simulink model "stepRecovery_compatibility"  (Simulink 8.3)
settings: Solver=ode3  SolverMode=SingleTasking  StartTime=0.0  StopTime="CONFIG.SIMULATION_TIME "  FixedStep=CONFIG.Ts  RelTol=1e-3
InitFcn:
  | cd(fileparts(which(bdroot)));
  | initStepRecovery;
values from neighbouring files (symbols this model uses):
  baseToWorldRotationPort = '/matlabTorqueBalancing/floatingBaseRotationMatrix:i'    [esperimento_fake2.mat]    (also in initStepRecovery.m = ['/' WBT_modelName '/floatingBaseRotationMatrix:i']; initTorqueBalancing.m = ['/' WBT_modelName '/floatingBaseRotationMatrix:i']; secondo_risultato.mat)
  bVectorConstraints = [0 0 0 0 0 0 0 0 0 0 0 0 ... (19 elements, 19x1)]    [esperimento_fake2.mat]    (also in secondo_risultato.mat)
  CONFIG =     [esperimento_fake2.mat]    (also in secondo_risultato.mat)
  ConstraintsMatrix = [3.73205080757 1 0.267949192431 -0.267949192431 -1 -3.73205080757 -3.73205080757 -1 -0.267949192431 0.267949192431 1 3.73205080757 ... (114 elements, 19x6)]    [esperimento_fake2.mat]    (also in secondo_risultato.mat)
  gain =     [esperimento_fake2.mat]    (also in secondo_risultato.mat)
  references =     [esperimento_fake2.mat]    (also in secondo_risultato.mat)
  reg =     [esperimento_fake2.mat]    (also in secondo_risultato.mat)
  ROBOT_DOF = 23    [esperimento_fake2.mat]    (also in secondo_risultato.mat)
  ROBOT_DOF_FOR_SIMULINK = [1 0 0 0 0 0 0 0 0 0 0 0 ... (529 elements, 23x23)]    [esperimento_fake2.mat]    (also in secondo_risultato.mat)
  sat =     [esperimento_fake2.mat]    (also in secondo_risultato.mat)
  SM =     [esperimento_fake2.mat]    (also in secondo_risultato.mat)
  sm =     [esperimento_fake2.mat]    (also in secondo_risultato.mat)
  WBT_modelName = 'matlabTorqueBalancing'    [esperimento_fake2.mat]    (also in initStepRecovery.m; initTorqueBalancing.m; secondo_risultato.mat)
  WBT_robotName = ''    [esperimento_fake2.mat]    (also in secondo_risultato.mat)
undefined symbols (not defined in the file or in its folder): bVectorConstraintsMPC, ConstraintsMatrixMPC, DiscIntNeverNeededParam, mpc_init
libraries: WBToolboxLibrary x191, simulink x22, simulink_extras x4
(part 4 of 6)

== system stepRecovery_compatibility/DesValues/State Machine/visualise inertial/w_H_root_link4 ==
  qj : Inport
  inertial : Inport  Port=2
  "CoM6D ->  CoMXYZ1" : Selector  NumberOfDimensions=2  InputPortWidth=7  IndexOptions=Index vector (dialog),Index vector (dialog)  Indices=[1 2 3],[1 2 3]  OutputSizes=1,1
  Constant : Constant  Value=zeros(3,1)
  Constant2 : Constant  Value=eye(4)
  Constant5 : Constant  Value=eye(4)
  Constant6 : Constant  Value=eye(4)
  Gain : Gain  Gain=pi/180
  Head state : WBToolboxLibrary/Utilities/Yarp Read  portName=[WBT_robotName, '/head/state:o']  signalSize=6  blocking=off  timestamp=off  autoconnect=on  errorOnConnection=off
  Inv\* : Product  Inputs=/*  Multiplication=Matrix(*)
  Inv\*1 : Product  Inputs=/*  Multiplication=Matrix(*)
  Inv\*2 : Product  Inputs=/  Multiplication=Matrix(*)
  Product : Product  Multiplication=Matrix(*)
  Selector : Selector  InputPortWidth=12  IndexOptions=Index vector (dialog)  Indices=[4 5 6 ]  OutputSizes=1
  Selector1 : Selector  InputPortWidth=6  IndexOptions=Index vector (dialog)  Indices=[1:3]  OutputSizes=1
  Switch : Switch  Criteria=u2 > Threshold
  Switch6 : Switch  Criteria=u2 > Threshold
  USE_IMU4EST_BASE : Constant  Value=CONFIG.USE_IMU4EST_BASE
  USE_IMU4EST_BASE1 : Constant  Value=CONFIG.CORRECT_NECK_IMU
  fromImuToHomogeousTransformFCN : MATLAB Function  TreatAsAtomicUnit=on
      settings: PermitHierarchicalResolution=ParametersOnly
  holder 1 : WBToolboxLibrary/Utilities/holder 
  holder 2 : WBToolboxLibrary/Utilities/holder 
  imu : WBToolboxLibrary/wholeBodyModel/Kinematics/Forward Kinematics  frameName='imu_frame'  robotName=WBT_robotName  localName=WBT_modelName  wbiFile=WBT_wbiFilename  wbiList=WBT_wbiList
  l_sole_acc : Scope
      settings: TimeRange=60  ShowLegends=on  MaxDataPoints=5000  SaveToWorkspace=off  YMin=-4.47309  YMax=14.2668  SampleTime=-1
  link : WBToolboxLibrary/wholeBodyModel/Kinematics/Forward Kinematics  frameName=link_name  robotName=WBT_robotName  localName=WBT_modelName  wbiFile=WBT_wbiFilename  wbiList=WBT_wbiList
  root_link : WBToolboxLibrary/wholeBodyModel/Kinematics/Forward Kinematics  frameName='root_link'  robotName=WBT_robotName  localName=WBT_modelName  wbiFile=WBT_wbiFilename  wbiList=WBT_wbiList
  w_H_root : Outport
  wires:
  Constant5/1 -> imu/1
  Inv\*/1 -> Inv\*2/1, holder 1/1, fromImuToHomogeousTransformFCN/1(imu_H_link)  "imu_H_link"
  imu/1 -> Inv\*/1
  Constant6/1 -> link/1
  Inv\*1/1 -> Switch6/3, fromImuToHomogeousTransformFCN/3(link_H_root)  "link_H_root"
  link/1 -> Inv\*/2, Inv\*1/1
  inertial/1 -> Selector/1, holder 2/1, fromImuToHomogeousTransformFCN/5(inertial)
  Switch6/1 -> w_H_root/1
  USE_IMU4EST_BASE/1 -> Switch6/2
  fromImuToHomogeousTransformFCN/1(w_H_root) -> Switch6/1
  Constant2/1 -> root_link/1
  qj/1 -> root_link/2, link/2, imu/2
  root_link/1 -> Inv\*1/2
  holder 1/1 -> fromImuToHomogeousTransformFCN/2(imu_H_link_0)
  holder 2/1 -> fromImuToHomogeousTransformFCN/4(inertial_0)
  Inv\*2/1 -> "CoM6D ->  CoMXYZ1"/1
  "CoM6D ->  CoMXYZ1"/1 -> Product/1  "l_sole_R_imu"
  Selector/1 -> Product/2  "imu_acce"
  Product/1 -> l_sole_acc/1
  Head state/1 -> Gain/1
  Selector1/1 -> Switch/1  "neck"
  USE_IMU4EST_BASE1/1 -> Switch/2
  Switch/1 -> fromImuToHomogeousTransformFCN/6(neck)
  Gain/1 -> Selector1/1
  Constant/1 -> Switch/3

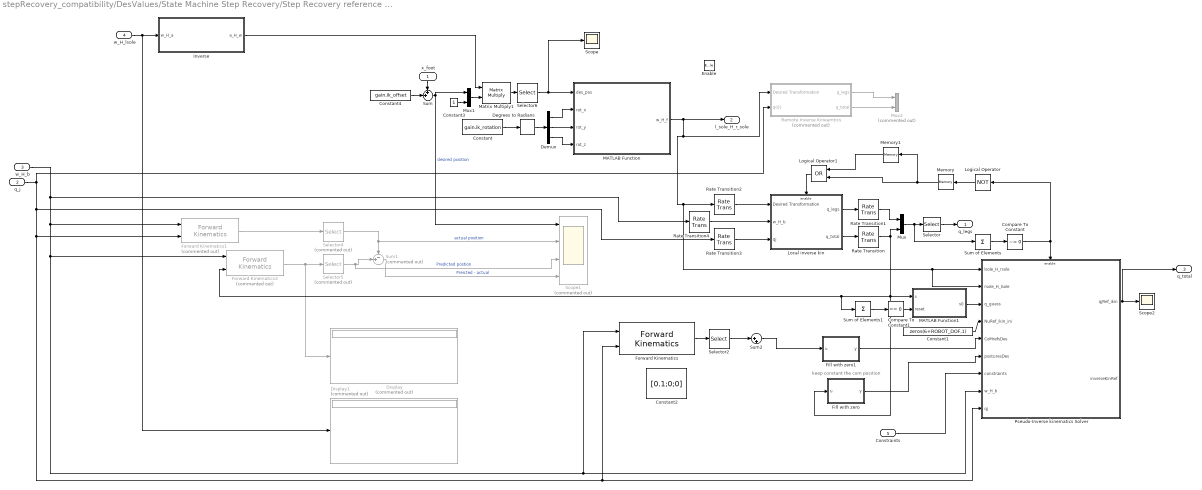
== system stepRecovery_compatibility/DesValues/State Machine Step Recovery/Step Recovery reference generator/Inverse Kinematics ==
  note: keep constant the com position
  x_foot : Inport
  q_j : Inport  Port=2
  w_H_b : Inport  Port=3
  w_H_lsole : Inport  Port=4
  Constraints : Inport  Port=5
  Enable : EnablePort
  Compare To Constant : simulink/Logic and Bit Operations/Compare To Constant  relop=~=  const=0  OutDataTypeStr=boolean
  Compare To Constant1 : simulink/Logic and Bit Operations/Compare To Constant  relop===  const=0  OutDataTypeStr=boolean
  Constant : Constant  Value=gain.ik_rotation
  Constant1 : Constant  Value=zeros(6+ROBOT_DOF,1)
  Constant2 : Constant  Value=[0.1;0;0]
  Constant3 : Constant
  Constant4 : Constant  Value=gain.ik_offset
  Degrees to Radians : simulink_extras/Transformations/Degrees to Radians
  Demux : Demux  Outputs=3
  Display : Display  Commented=on
  Display1 : Display  Commented=on
  Fill with zero : MATLAB Function  TreatAsAtomicUnit=on
      settings: PermitHierarchicalResolution=ParametersOnly
  Fill with zero1 : MATLAB Function  TreatAsAtomicUnit=on
      settings: PermitHierarchicalResolution=ParametersOnly
  Forward Kinematics : WBToolboxLibrary/wholeBodyModel/Kinematics/Forward Kinematics  frameName='com'  robotName=WBT_robotName  localName=WBT_modelName  wbiFile=WBT_wbiFilename  wbiList=WBT_wbiList
  Forward Kinematics1 : WBToolboxLibrary/wholeBodyModel/Kinematics/Forward Kinematics  Commented=on  frameName='r_sole'  robotName=WBT_robotName  localName=WBT_modelName  wbiFile=WBT_wbiFilename  wbiList=WBT_wbiList
  Forward Kinematics3 : WBToolboxLibrary/wholeBodyModel/Kinematics/Forward Kinematics  Commented=on  frameName='r_sole'  robotName=WBT_robotName  localName=WBT_modelName  wbiFile=WBT_wbiFilename  wbiList=WBT_wbiList
  Inverse : MATLAB Function  TreatAsAtomicUnit=on
      settings: PermitHierarchicalResolution=ParametersOnly
  Local inverse kin : Subsystem  TreatAsAtomicUnit=on  SystemSampleTime=CONFIG.Ts*5
  Logical Operator : Logic  Operator=NOT  AllPortsSameDT=off  OutDataTypeStr=boolean
  Logical Operator1 : Logic  Operator=OR  AllPortsSameDT=off  OutDataTypeStr=boolean
  MATLAB Function : MATLAB Function  TreatAsAtomicUnit=on
      settings: PermitHierarchicalResolution=ParametersOnly
  MATLAB Function1 : MATLAB Function  TreatAsAtomicUnit=on
      settings: PermitHierarchicalResolution=ParametersOnly
  Matrix Multiply1 : Product  Multiplication=Matrix(*)
  Memory : Memory  X0=1
  Memory1 : Memory  X0=1
  Mux : Mux  Inputs=2
  Mux1 : Mux  Inputs=2
  Mux2 : Mux  Commented=on  Inputs=2
  Pseudo-Inverse kinematics Solver : Subsystem
  Rate Transition{,1..4} (5 alike) : RateTransition
  Remote Inverse Kineamtics : Subsystem  Commented=on
  Scope : Scope
      settings: TimeRange=auto  MaxDataPoints=5000  SaveToWorkspace=off  YMin=-0.33081  YMax=0.15171  SampleTime=-1
  Scope1 : Scope  Commented=on  NumInputPorts=4
      settings: TimeRange=auto  LimitDataPoints=on  MaxDataPoints=5000  SaveToWorkspace=off  SaveName=ScopeData2  YMin=-0.12177~-0.3226~-0.20619~-0.23804  YMax=0.12942~0.28839~0.2954~0.28029  SampleTime=-1  DataFormat=Array
  Scope2 : Scope
      settings: TimeRange=auto  MaxDataPoints=5000  SaveToWorkspace=off  YMin=-1.24723  YMax=2.00344  SampleTime=-1
  Selector : Selector  InputPortWidth=12+23  IndexOptions=Index vector (dialog)  Indices=[1:12]  OutputSizes=1
  Selector2 : Selector  NumberOfDimensions=2  InputPortWidth=3  IndexOptions=Index vector (dialog),Index vector (dialog)  Indices=[1:3],4  OutputSizes=1,1
  Selector4 : Selector  Commented=on  NumberOfDimensions=2  InputPortWidth=4  IndexOptions=Index vector (dialog),Index vector (dialog)  Indices=[1:3],4  OutputSizes=1,1
  Selector5 : Selector  Commented=on  NumberOfDimensions=2  InputPortWidth=4  IndexOptions=Index vector (dialog),Index vector (dialog)  Indices=[1:3],4  OutputSizes=1,1
  Selector6 : Selector  InputPortWidth=4  IndexOptions=Index vector (dialog)  Indices=[1:3]  OutputSizes=1
  Sum : Sum  Inputs=++|
  Sum of Elements : Sum  Inputs=+
  Sum of Elements1 : Sum  Inputs=+
  Sum1 : Sum  Commented=on  Inputs=-+|
  Sum2 : Sum  Inputs=|++
  q_legs : Outport
  l_sole_H_r_sole : Outport  Port=2
  "q_total " : Outport  Port=3
  wires:
  w_H_b/1 -> Forward Kinematics1/1, Forward Kinematics/1, Pseudo-Inverse kinematics Solver/8("w_H_b "), Forward Kinematics3/1, Rate Transition4/1
  MATLAB Function/1(w_H_f) -> l_sole_H_r_sole/1, Pseudo-Inverse kinematics Solver/2(rsole_H_lsole), Pseudo-Inverse kinematics Solver/1("lsole_H_rsole "), Rate Transition2/1, Remote Inverse Kineamtics/1(Desired Transformation)
  w_H_lsole/1 -> Display1/1, Inverse/1(w_H_a)
  Inverse/1(a_H_w) -> Matrix Multiply1/1
  Forward Kinematics1/1 -> Selector4/1
  Sum/1 -> Mux1/1, Scope1/1  "desired position"
  Constant4/1 -> Sum/2
  x_foot/1 -> Sum/1
  Forward Kinematics3/1 -> Display/1, Selector5/1
  Selector4/1 -> Sum1/1, Scope1/2  "actual position"
  Sum1/1 -> Scope1/4  "Preicted - actual"
  Mux1/1 -> Matrix Multiply1/2
  Constant3/1 -> Mux1/2
  Selector6/1 -> Scope/1, MATLAB Function/1(des_pos)
  Matrix Multiply1/1 -> Selector6/1
  Selector5/1 -> Scope1/3, Sum1/2  "Predicted postion"
  Local inverse kin/2("q_total ") -> Rate Transition/1
  Constant/1 -> Degrees to Radians/1
  Degrees to Radians/1 -> Demux/1
  Demux/2 -> MATLAB Function/3(rot_y)
  Demux/1 -> MATLAB Function/2(rot_x)
  Demux/3 -> MATLAB Function/4(rot_z)
  Local inverse kin/1(q_legs) -> Rate Transition1/1
  Selector/1 -> q_legs/1
  Mux/1 -> Sum of Elements/1, Selector/1
  Remote Inverse Kineamtics/1(q_legs) -> Mux2/1
  Remote Inverse Kineamtics/2(q_total) -> Mux2/2
  Rate Transition1/1 -> Mux/1
  Rate Transition2/1 -> Local inverse kin/1(Desired Transformation)
  Rate Transition3/1 -> Local inverse kin/3(qj)
  Rate Transition4/1 -> Local inverse kin/2(w_H_b)
  Constant1/1 -> Pseudo-Inverse kinematics Solver/4(NuRef_ikin_ini)
  Constraints/1 -> Pseudo-Inverse kinematics Solver/7(constraints)
  Fill with zero1/1(y) -> Pseudo-Inverse kinematics Solver/5(CoMrefsDes)
  Forward Kinematics/1 -> Selector2/1
  q_j/1 -> Remote Inverse Kineamtics/2(q(0)), Forward Kinematics/2, Pseudo-Inverse kinematics Solver/9(qj), Forward Kinematics1/2, Rate Transition3/1
  Sum2/1 -> Fill with zero1/1(u)
  Fill with zero/1(y) -> Pseudo-Inverse kinematics Solver/6(posturesDes)
  Rate Transition/1 -> Fill with zero/1(u), MATLAB Function1/1(s), Sum of Elements1/1, Forward Kinematics3/2, Mux/2
  Pseudo-Inverse kinematics Solver/1(qjRef_ikin) -> Scope2/1, "q_total "/1
  Sum of Elements/1 -> Compare To Constant/1
  MATLAB Function1/1(s0) -> Pseudo-Inverse kinematics Solver/3(q_guess)
  Sum of Elements1/1 -> Compare To Constant1/1
  Compare To Constant1/1 -> MATLAB Function1/2(reset)
  Logical Operator/1 -> Memory/1
  Compare To Constant/1 -> Pseudo-Inverse kinematics Solver/Enable, Logical Operator/1
  Memory/1 -> Memory1/1, Logical Operator1/2
  Memory1/1 -> Logical Operator1/1
  Logical Operator1/1 -> Local inverse kin/Enable
  Selector2/1 -> Sum2/1

== system stepRecovery_compatibility/DesValues/State Machine Step Recovery/Step Recovery reference generator/Selector and Saturation ==
  CP : Inport
  FPE : Inport  Port=2
  "CP1 " : Inport  Port=3
  Constant : Constant  Value=2*sqrt(gain.leg_length^2 - gain.minimum_height^2)
  Constant1 : Constant  Value=gain.min_step_length
  Constant2 : Constant  Value=CONFIG.SR.TECHNIQUE
  Demux : Demux
  Dot Product : DotProduct  InputSameDT=on  OutDataTypeStr=Inherit: Inherit via internal rule
  MATLAB Function : MATLAB Function  TreatAsAtomicUnit=on
      settings: PermitHierarchicalResolution=ParametersOnly
  Multiport Switch : MultiPortSwitch  DataPortOrder=Specify indices  DataPortIndices={2,1,0}
  Mux : Mux  Inputs=3
  Mux1 : Mux  Inputs=3
  Scope : Scope  Commented=on  NumInputPorts=4
      settings: TimeRange=auto  MaxDataPoints=5000  SaveToWorkspace=off  SaveName=ScopeData2  YMin=-1.125~-0.12972~-0.45531~-0.45531  YMax=0.125~1.16911~0.52006~0.52006  SampleTime=-1
  Sqrt : Sqrt  SaturateOnIntegerOverflow=on
  To Workspace : ToWorkspace  VariableName=IS_SATURATED  SampleTime=-1
      settings: Save2DSignal=2-D array (concatenate along first dimension)
  STEP : Outport
  x_sat : Outport  Port=2
  wires:
  Mux1/1 -> Scope/4, Dot Product/2, Dot Product/1, MATLAB Function/1(x)  "X"
  Constant/1 -> MATLAB Function/2(max_d), Mux/2  "max module"
  MATLAB Function/1(x_sat) -> Scope/3, x_sat/1  "X_SAT"
  MATLAB Function/2(SAT) -> Scope/1, To Workspace/1  "SAT"
  Mux/1 -> Scope/2  "MODULE"
  Sqrt/1 -> Mux/1  "desired module"
  Dot Product/1 -> Sqrt/1
  Constant1/1 -> Mux/3, MATLAB Function/3(min_d)  "min module"
  Multiport Switch/1 -> Demux/1  "X"
  Demux/4 -> STEP/1
  CP/1 -> Multiport Switch/4  "X"
  FPE/1 -> Multiport Switch/3
  "CP1 "/1 -> Multiport Switch/2
  Constant2/1 -> Multiport Switch/1
  Demux/2 -> Mux1/2
  Demux/3 -> Mux1/3
  Demux/1 -> Mux1/1  "X"

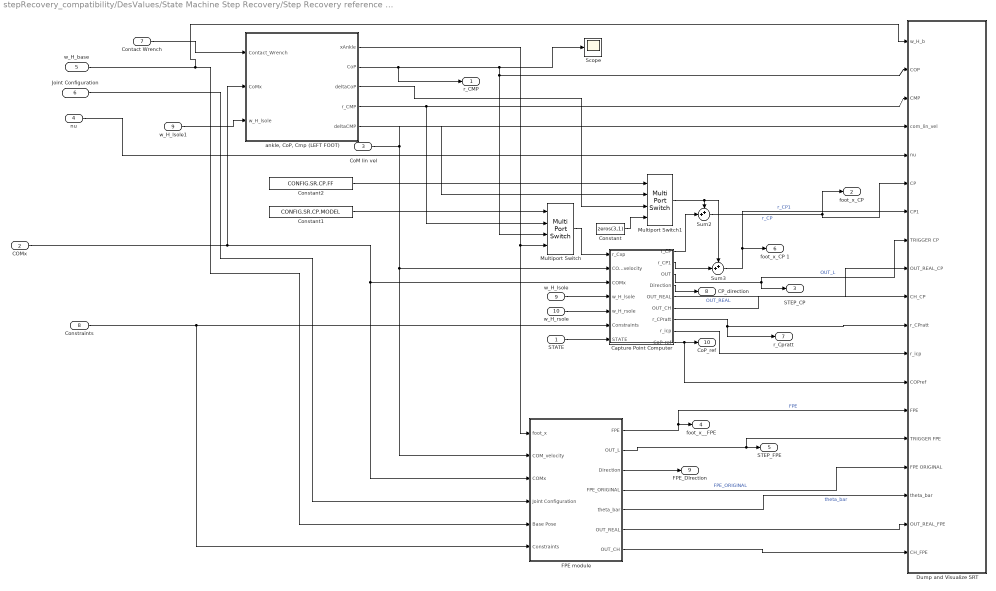
== system stepRecovery_compatibility/DesValues/State Machine Step Recovery/Step Recovery reference generator/Step Recovery Techniques  ==
  STATE : Inport
  COMx : Inport  Port=2
  CoM lin vel : Inport  Port=3
  nu : Inport  Port=4
  w_H_base : Inport  Port=5
  Joint Configuration : Inport  Port=6
  Contact Wrench : Inport  Port=7
  "Constraints " : Inport  Port=8
  w_H_lsole : Inport  Port=9
  w_H_rsole : Inport  Port=10
  Capture Point Computer : Subsystem
  Constant : Constant  Value=zeros(3,1)
  Constant1 : Constant  Value=CONFIG.SR.CP.MODEL
  Constant2 : Constant  Value=CONFIG.SR.CP.FF
  "Dump and Visualize SRT " : Subsystem
  FPE module : Subsystem
  Multiport Switch : MultiPortSwitch  DataPortOrder=Specify indices  DataPortIndices={2,1,0}
  Multiport Switch1 : MultiPortSwitch  DataPortOrder=Specify indices  DataPortIndices={2,1,0}
  Scope : Scope
      settings: TimeRange=auto  MaxDataPoints=5000  SaveToWorkspace=off  SaveName=ScopeData2  YMin=-0.03977  YMax=0.14577  SampleTime=-1
  Sum2 : Sum  Inputs=++|
  Sum3 : Sum  Inputs=++|
  "ankle, CoP, Cmp (LEFT FOOT)" : Subsystem
  w_H_lsole1 : InportShadow  Port=9
  r_CMP : Outport
  "foot_x_CP " : Outport  Port=2
  STEP_CP : Outport  Port=3
  foot_x__FPE : Outport  Port=4
  STEP_FPE : Outport  Port=5
  foot_x_CP 1 : Outport  Port=6
  "r_Cpratt " : Outport  Port=7
  CP_direction : Outport  Port=8
  FPE_DIrection : Outport  Port=9
  "CoP_ref " : Outport  Port=10
  wires:
  Joint Configuration/1 -> FPE module/4(Joint Configuration)
  w_H_base/1 -> FPE module/5(Base Pose), "Dump and Visualize SRT "/1(w_H_b)
  FPE module/1(FPE) -> "Dump and Visualize SRT "/14(FPE), foot_x__FPE/1  "FPE"
  Sum2/1 -> "foot_x_CP "/1, "Dump and Visualize SRT "/6(CP)  "r_CP"
  Capture Point Computer/3(OUT) -> "Dump and Visualize SRT "/8(TRIGGER CP), STEP_CP/1  "OUT_L"
  Sum3/1 -> "Dump and Visualize SRT "/7(CP1), foot_x_CP 1/1  "r_CP1"
  FPE module/3(Direction) -> FPE_DIrection/1
  Capture Point Computer/4(Direction) -> CP_direction/1
  Capture Point Computer/1(r_CP) -> Sum2/2
  Capture Point Computer/2(r_CP1) -> Sum3/2
  "Constraints "/1 -> FPE module/6(Constraints), Capture Point Computer/6("Constraints ")
  FPE module/2(OUT_L) -> "Dump and Visualize SRT "/15(TRIGGER FPE), STEP_FPE/1
  CoM lin vel/1 -> "Dump and Visualize SRT "/4(com_lin_vel), FPE module/2(COM_velocity), Capture Point Computer/2(COM velocity)
  COMx/1 -> FPE module/3(COMx), Capture Point Computer/3(COMx), "ankle, CoP, Cmp (LEFT FOOT)"/2(CoMx)
  "ankle, CoP, Cmp (LEFT FOOT)"/2(CoP) -> r_CMP/1, Scope/1, Multiport Switch/3, "Dump and Visualize SRT "/2(COP)
  "ankle, CoP, Cmp (LEFT FOOT)"/1(xAnkle) -> FPE module/1(foot_x), Multiport Switch/4
  Contact Wrench/1 -> "ankle, CoP, Cmp (LEFT FOOT)"/1(Contact_Wrench)
  nu/1 -> "Dump and Visualize SRT "/5(nu)
  "ankle, CoP, Cmp (LEFT FOOT)"/4(r_CMP) -> "Dump and Visualize SRT "/3(CMP), Multiport Switch/2
  Capture Point Computer/5(OUT_REAL) -> "Dump and Visualize SRT "/9(OUT_REAL_CP)  "OUT_REAL"
  Capture Point Computer/6(OUT_CH) -> "Dump and Visualize SRT "/10(CH_CP)
  FPE module/4(FPE_ORIGINAL) -> "Dump and Visualize SRT "/16(FPE ORIGINAL)  "FPE_ORIGINAL"
  FPE module/5(theta_bar) -> "Dump and Visualize SRT "/17(theta_bar)  "theta_bar"
  FPE module/6(OUT_REAL) -> "Dump and Visualize SRT "/18(OUT_REAL_FPE)
  FPE module/7(OUT_CH) -> "Dump and Visualize SRT "/19(CH_FPE)
  Multiport Switch/1 -> Capture Point Computer/1(r_Cxp)
  Multiport Switch1/1 -> Sum3/1, Sum2/1
  Constant/1 -> Multiport Switch1/4
  "ankle, CoP, Cmp (LEFT FOOT)"/3(deltaCoP) -> Multiport Switch1/3
  "ankle, CoP, Cmp (LEFT FOOT)"/5(deltaCMP) -> Multiport Switch1/2
  Constant1/1 -> Multiport Switch/1
  Constant2/1 -> Multiport Switch1/1
  w_H_lsole/1 -> Capture Point Computer/4(w_H_lsole)
  w_H_rsole/1 -> Capture Point Computer/5(w_H_rsole)
  w_H_lsole1/1 -> "ankle, CoP, Cmp (LEFT FOOT)"/3(w_H_lsole)
  STATE/1 -> Capture Point Computer/7(STATE)
  Capture Point Computer/7("r_CPratt ") -> "r_Cpratt "/1, "Dump and Visualize SRT "/11("r_CPratt ")
  Capture Point Computer/8(r_icp) -> "Dump and Visualize SRT "/12(r_icp)
  Capture Point Computer/9(CoP_ref) -> "Dump and Visualize SRT "/13(COPref), "CoP_ref "/1

== system stepRecovery_compatibility/DesValues/State Machine Step Recovery/visualise inertial/Visualize hom transf1 ==
  H : Inport
  "CoM6D ->  CoMXYZ1" : Selector  NumberOfDimensions=2  InputPortWidth=7  IndexOptions=Index vector (dialog),Index vector (dialog)  Indices=[1 2 3],[1 2 3]  OutputSizes=1,1
  "CoM6D ->  CoMXYZ2" : Selector  NumberOfDimensions=2  InputPortWidth=7  IndexOptions=Index vector (dialog),Index vector (dialog)  Indices=[1 2 3],[4]  OutputSizes=1,1
  Hom : Scope
      settings: TimeRange=auto  ShowLegends=on  MaxDataPoints=5000  SaveToWorkspace=off  SaveName=ScopeData3  YMin=-0.02533  YMax=0.01393  SampleTime=-1
  MATLAB Function : MATLAB Function  TreatAsAtomicUnit=on
      settings: PermitHierarchicalResolution=ParametersOnly
  p : Scope
      settings: TimeRange=auto  MaxDataPoints=5000  SaveToWorkspace=off  SaveName=ScopeData2  YMin=-0.05005  YMax=0.09732  SampleTime=-1
  rollPitchYaw : Scope
      settings: TimeRange=auto  ShowLegends=on  MaxDataPoints=5000  SaveToWorkspace=off  YMin=-0.15453  YMax=0.04472  SampleTime=-1
  wires:
  MATLAB Function/1(rollPitchYaw) -> rollPitchYaw/1
  "CoM6D ->  CoMXYZ1"/1 -> MATLAB Function/1(R)
  H/1 -> "CoM6D ->  CoMXYZ1"/1, Hom/1, "CoM6D ->  CoMXYZ2"/1
  "CoM6D ->  CoMXYZ2"/1 -> p/1

== system stepRecovery_compatibility/DesValues/State Machine Step Recovery/visualise inertial/Visualize hom transf2 ==
  H : Inport
  "CoM6D ->  CoMXYZ1" : Selector  NumberOfDimensions=2  InputPortWidth=7  IndexOptions=Index vector (dialog),Index vector (dialog)  Indices=[1 2 3],[1 2 3]  OutputSizes=1,1
  "CoM6D ->  CoMXYZ2" : Selector  NumberOfDimensions=2  InputPortWidth=7  IndexOptions=Index vector (dialog),Index vector (dialog)  Indices=[1 2 3],[4]  OutputSizes=1,1
  Hom : Scope
      settings: TimeRange=auto  ShowLegends=on  MaxDataPoints=5000  SaveToWorkspace=off  SaveName=ScopeData3  YMin=-0.02533  YMax=0.01393  SampleTime=-1
  MATLAB Function : MATLAB Function  TreatAsAtomicUnit=on
      settings: PermitHierarchicalResolution=ParametersOnly
  p : Scope
      settings: TimeRange=auto  MaxDataPoints=5000  SaveToWorkspace=off  SaveName=ScopeData2  YMin=-0.05005  YMax=0.09732  SampleTime=-1
  rollPitchYaw : Scope
      settings: TimeRange=auto  ShowLegends=on  MaxDataPoints=5000  SaveToWorkspace=off  YMin=-0.15453  YMax=0.04472  SampleTime=-1
  wires:
  MATLAB Function/1(rollPitchYaw) -> rollPitchYaw/1
  "CoM6D ->  CoMXYZ1"/1 -> MATLAB Function/1(R)
  H/1 -> "CoM6D ->  CoMXYZ1"/1, Hom/1, "CoM6D ->  CoMXYZ2"/1
  "CoM6D ->  CoMXYZ2"/1 -> p/1

== system stepRecovery_compatibility/DesValues/State Machine Step Recovery/visualise inertial/Visualize hom transf3 ==
  H : Inport
  "CoM6D ->  CoMXYZ1" : Selector  NumberOfDimensions=2  InputPortWidth=7  IndexOptions=Index vector (dialog),Index vector (dialog)  Indices=[1 2 3],[1 2 3]  OutputSizes=1,1
  "CoM6D ->  CoMXYZ2" : Selector  NumberOfDimensions=2  InputPortWidth=7  IndexOptions=Index vector (dialog),Index vector (dialog)  Indices=[1 2 3],[4]  OutputSizes=1,1
  Hom : Scope
      settings: TimeRange=auto  ShowLegends=on  MaxDataPoints=5000  SaveToWorkspace=off  SaveName=ScopeData3  YMin=-0.02533  YMax=0.01393  SampleTime=-1
  MATLAB Function : MATLAB Function  TreatAsAtomicUnit=on
      settings: PermitHierarchicalResolution=ParametersOnly
  p : Scope
      settings: TimeRange=auto  MaxDataPoints=5000  SaveToWorkspace=off  SaveName=ScopeData2  YMin=-0.05005  YMax=0.09732  SampleTime=-1
  rollPitchYaw : Scope
      settings: TimeRange=auto  ShowLegends=on  MaxDataPoints=5000  SaveToWorkspace=off  YMin=-0.15453  YMax=0.04472  SampleTime=-1
  wires:
  MATLAB Function/1(rollPitchYaw) -> rollPitchYaw/1
  "CoM6D ->  CoMXYZ1"/1 -> MATLAB Function/1(R)
  H/1 -> "CoM6D ->  CoMXYZ1"/1, Hom/1, "CoM6D ->  CoMXYZ2"/1
  "CoM6D ->  CoMXYZ2"/1 -> p/1

== system stepRecovery_compatibility/DesValues/State Machine Step Recovery/visualise inertial/Visualize hom transf4 ==
  H : Inport
  "CoM6D ->  CoMXYZ1" : Selector  NumberOfDimensions=2  InputPortWidth=7  IndexOptions=Index vector (dialog),Index vector (dialog)  Indices=[1 2 3],[1 2 3]  OutputSizes=1,1
  "CoM6D ->  CoMXYZ2" : Selector  NumberOfDimensions=2  InputPortWidth=7  IndexOptions=Index vector (dialog),Index vector (dialog)  Indices=[1 2 3],[4]  OutputSizes=1,1
  Hom : Scope
      settings: TimeRange=auto  ShowLegends=on  MaxDataPoints=5000  SaveToWorkspace=off  SaveName=ScopeData3  YMin=-0.02533  YMax=0.01393  SampleTime=-1
  MATLAB Function : MATLAB Function  TreatAsAtomicUnit=on
      settings: PermitHierarchicalResolution=ParametersOnly
  p : Scope
      settings: TimeRange=auto  MaxDataPoints=5000  SaveToWorkspace=off  SaveName=ScopeData2  YMin=-0.05005  YMax=0.09732  SampleTime=-1
  rollPitchYaw : Scope
      settings: TimeRange=auto  ShowLegends=on  MaxDataPoints=5000  SaveToWorkspace=off  YMin=-0.15453  YMax=0.04472  SampleTime=-1
  wires:
  MATLAB Function/1(rollPitchYaw) -> rollPitchYaw/1
  "CoM6D ->  CoMXYZ1"/1 -> MATLAB Function/1(R)
  H/1 -> "CoM6D ->  CoMXYZ1"/1, Hom/1, "CoM6D ->  CoMXYZ2"/1
  "CoM6D ->  CoMXYZ2"/1 -> p/1

== system stepRecovery_compatibility/DesValues/State Machine Step Recovery/visualise inertial/Visualize hom transf5 ==
  H : Inport
  "CoM6D ->  CoMXYZ1" : Selector  NumberOfDimensions=2  InputPortWidth=7  IndexOptions=Index vector (dialog),Index vector (dialog)  Indices=[1 2 3],[1 2 3]  OutputSizes=1,1
  Hom : Scope
      settings: TimeRange=auto  ShowLegends=on  MaxDataPoints=5000  SaveToWorkspace=off  SaveName=ScopeData3  YMin=-0.02533  YMax=0.01393  SampleTime=-1
  MATLAB Function : MATLAB Function  TreatAsAtomicUnit=on
      settings: PermitHierarchicalResolution=ParametersOnly
  p : Scope
      settings: TimeRange=auto  ShowLegends=on  MaxDataPoints=5000  SaveToWorkspace=off  SaveName=ScopeData2  YMin=-0.04515  YMax=0.14859  SampleTime=-1
  position : Selector  NumberOfDimensions=2  InputPortWidth=7  IndexOptions=Index vector (dialog),Index vector (dialog)  Indices=[1 2 3],[4]  OutputSizes=1,1
  rollPitchYaw : Scope
      settings: TimeRange=auto  ShowLegends=on  MaxDataPoints=5000  SaveToWorkspace=off  YMin=-3.6963  YMax=1.91309  SampleTime=-1
  wires:
  MATLAB Function/1(rollPitchYaw) -> rollPitchYaw/1  "rollPitchYaw"
  "CoM6D ->  CoMXYZ1"/1 -> MATLAB Function/1(R)
  H/1 -> "CoM6D ->  CoMXYZ1"/1, Hom/1, position/1  "H"
  position/1 -> p/1  "position"

== system stepRecovery_compatibility/DesValues/State Machine Step Recovery/visualise inertial/Visualize hom transf6 ==
  H : Inport
  "CoM6D ->  CoMXYZ1" : Selector  NumberOfDimensions=2  InputPortWidth=7  IndexOptions=Index vector (dialog),Index vector (dialog)  Indices=[1 2 3],[1 2 3]  OutputSizes=1,1
  "CoM6D ->  CoMXYZ2" : Selector  NumberOfDimensions=2  InputPortWidth=7  IndexOptions=Index vector (dialog),Index vector (dialog)  Indices=[1 2 3],[4]  OutputSizes=1,1
  Hom : Scope
      settings: TimeRange=auto  ShowLegends=on  MaxDataPoints=5000  SaveToWorkspace=off  SaveName=ScopeData3  YMin=-0.02533  YMax=0.01393  SampleTime=-1
  MATLAB Function : MATLAB Function  TreatAsAtomicUnit=on
      settings: PermitHierarchicalResolution=ParametersOnly
  p : Scope
      settings: TimeRange=auto  MaxDataPoints=5000  SaveToWorkspace=off  SaveName=ScopeData2  YMin=-0.05005  YMax=0.09732  SampleTime=-1
  rollPitchYaw : Scope
      settings: TimeRange=auto  ShowLegends=on  MaxDataPoints=5000  SaveToWorkspace=off  YMin=-0.15453  YMax=0.04472  SampleTime=-1
  wires:
  MATLAB Function/1(rollPitchYaw) -> rollPitchYaw/1
  "CoM6D ->  CoMXYZ1"/1 -> MATLAB Function/1(R)
  H/1 -> "CoM6D ->  CoMXYZ1"/1, Hom/1, "CoM6D ->  CoMXYZ2"/1
  "CoM6D ->  CoMXYZ2"/1 -> p/1

== system stepRecovery_compatibility/DesValues/State Machine Step Recovery/visualise inertial/l_sole_H_root_link2 ==
  qj : Inport
  Constant5 : Constant  Value=eye(4)
  Constant6 : Constant  Value=eye(4)
  Inv\* : Product  Inputs=/*  Multiplication=Matrix(*)
  Visualize hom transf4 : Subsystem
  link_name : WBToolboxLibrary/wholeBodyModel/Kinematics/Forward Kinematics  frameName=link_name  robotName=WBT_robotName  localName=WBT_modelName  wbiFile=WBT_wbiFilename  wbiList=WBT_wbiList
  root_link : WBToolboxLibrary/wholeBodyModel/Kinematics/Forward Kinematics  frameName='root_link'  robotName=WBT_robotName  localName=WBT_modelName  wbiFile=WBT_wbiFilename  wbiList=WBT_wbiList
  link_name_H_root_link : Outport
  wires:
  root_link/1 -> Inv\*/2, Visualize hom transf4/1(H)
  qj/1 -> root_link/2, link_name/2
  Constant6/1 -> root_link/1
  link_name/1 -> Inv\*/1
  Inv\*/1 -> link_name_H_root_link/1  "link_name_H_root_link"
  Constant5/1 -> link_name/1

== system stepRecovery_compatibility/DesValues/State Machine Step Recovery/visualise inertial/l_sole_H_root_link3 ==
  qj : Inport
  Constant5 : Constant  Value=eye(4)
  Constant6 : Constant  Value=eye(4)
  Inv\* : Product  Inputs=/*  Multiplication=Matrix(*)
  Visualize hom transf4 : Subsystem
  link_name : WBToolboxLibrary/wholeBodyModel/Kinematics/Forward Kinematics  frameName=link_name  robotName=WBT_robotName  localName=WBT_modelName  wbiFile=WBT_wbiFilename  wbiList=WBT_wbiList
  root_link : WBToolboxLibrary/wholeBodyModel/Kinematics/Forward Kinematics  frameName='root_link'  robotName=WBT_robotName  localName=WBT_modelName  wbiFile=WBT_wbiFilename  wbiList=WBT_wbiList
  link_name_H_root_link : Outport
  wires:
  root_link/1 -> Inv\*/2, Visualize hom transf4/1(H)
  qj/1 -> root_link/2, link_name/2
  Constant6/1 -> root_link/1
  link_name/1 -> Inv\*/1
  Inv\*/1 -> link_name_H_root_link/1  "link_name_H_root_link"
  Constant5/1 -> link_name/1

== system stepRecovery_compatibility/DesValues/State Machine Step Recovery/visualise inertial/w_H_root_link1 ==
  qj : Inport
  inertial : Inport  Port=2
  "CoM6D ->  CoMXYZ1" : Selector  NumberOfDimensions=2  InputPortWidth=7  IndexOptions=Index vector (dialog),Index vector (dialog)  Indices=[1 2 3],[1 2 3]  OutputSizes=1,1
  Constant : Constant  Value=zeros(3,1)
  Constant2 : Constant  Value=eye(4)
  Constant5 : Constant  Value=eye(4)
  Constant6 : Constant  Value=eye(4)
  Gain : Gain  Gain=pi/180
  Head state : WBToolboxLibrary/Utilities/Yarp Read  portName=[WBT_robotName, '/head/state:o']  signalSize=6  blocking=off  timestamp=off  autoconnect=on  errorOnConnection=off
  Inv\* : Product  Inputs=/*  Multiplication=Matrix(*)
  Inv\*1 : Product  Inputs=/*  Multiplication=Matrix(*)
  Inv\*2 : Product  Inputs=/  Multiplication=Matrix(*)
  Product : Product  Multiplication=Matrix(*)
  Selector : Selector  InputPortWidth=12  IndexOptions=Index vector (dialog)  Indices=[4 5 6 ]  OutputSizes=1
  Selector1 : Selector  InputPortWidth=6  IndexOptions=Index vector (dialog)  Indices=[1:3]  OutputSizes=1
  Switch : Switch  Criteria=u2 > Threshold
  Switch6 : Switch  Criteria=u2 > Threshold
  USE_IMU4EST_BASE : Constant  Value=CONFIG.USE_IMU4EST_BASE
  USE_IMU4EST_BASE1 : Constant  Value=CONFIG.CORRECT_NECK_IMU
  fromImuToHomogeousTransformFCN : MATLAB Function  TreatAsAtomicUnit=on
      settings: PermitHierarchicalResolution=ParametersOnly
  holder 1 : WBToolboxLibrary/Utilities/holder 
  holder 2 : WBToolboxLibrary/Utilities/holder 
  imu : WBToolboxLibrary/wholeBodyModel/Kinematics/Forward Kinematics  frameName='imu_frame'  robotName=WBT_robotName  localName=WBT_modelName  wbiFile=WBT_wbiFilename  wbiList=WBT_wbiList
  l_sole_acc : Scope
      settings: TimeRange=60  ShowLegends=on  MaxDataPoints=5000  SaveToWorkspace=off  YMin=-4.47309  YMax=14.2668  SampleTime=-1
  link : WBToolboxLibrary/wholeBodyModel/Kinematics/Forward Kinematics  frameName=link_name  robotName=WBT_robotName  localName=WBT_modelName  wbiFile=WBT_wbiFilename  wbiList=WBT_wbiList
  root_link : WBToolboxLibrary/wholeBodyModel/Kinematics/Forward Kinematics  frameName='root_link'  robotName=WBT_robotName  localName=WBT_modelName  wbiFile=WBT_wbiFilename  wbiList=WBT_wbiList
  w_H_root : Outport
  wires:
  Constant/1 -> Switch/3
  Gain/1 -> Selector1/1
  Switch/1 -> fromImuToHomogeousTransformFCN/6(neck)
  USE_IMU4EST_BASE1/1 -> Switch/2
  Selector1/1 -> Switch/1  "neck"
  Head state/1 -> Gain/1
  Product/1 -> l_sole_acc/1
  Selector/1 -> Product/2  "imu_acce"
  "CoM6D ->  CoMXYZ1"/1 -> Product/1  "l_sole_R_imu"
  Inv\*2/1 -> "CoM6D ->  CoMXYZ1"/1
  holder 2/1 -> fromImuToHomogeousTransformFCN/4(inertial_0)
  holder 1/1 -> fromImuToHomogeousTransformFCN/2(imu_H_link_0)
  root_link/1 -> Inv\*1/2
  qj/1 -> imu/2, link/2, root_link/2
  Constant2/1 -> root_link/1
  fromImuToHomogeousTransformFCN/1(w_H_root) -> Switch6/1
  USE_IMU4EST_BASE/1 -> Switch6/2
  Switch6/1 -> w_H_root/1
  inertial/1 -> fromImuToHomogeousTransformFCN/5(inertial), holder 2/1, Selector/1
  link/1 -> Inv\*1/1, Inv\*/2
  Inv\*1/1 -> fromImuToHomogeousTransformFCN/3(link_H_root), Switch6/3  "link_H_root"
  Constant6/1 -> link/1
  imu/1 -> Inv\*/1
  Inv\*/1 -> fromImuToHomogeousTransformFCN/1(imu_H_link), holder 1/1, Inv\*2/1  "imu_H_link"
  Constant5/1 -> imu/1

== system stepRecovery_compatibility/DesValues/State Machine Step Recovery/visualise inertial/w_H_root_link4 ==
  qj : Inport
  inertial : Inport  Port=2
  "CoM6D ->  CoMXYZ1" : Selector  NumberOfDimensions=2  InputPortWidth=7  IndexOptions=Index vector (dialog),Index vector (dialog)  Indices=[1 2 3],[1 2 3]  OutputSizes=1,1
  Constant : Constant  Value=zeros(3,1)
  Constant2 : Constant  Value=eye(4)
  Constant5 : Constant  Value=eye(4)
  Constant6 : Constant  Value=eye(4)
  Gain : Gain  Gain=pi/180
  Head state : WBToolboxLibrary/Utilities/Yarp Read  portName=[WBT_robotName, '/head/state:o']  signalSize=6  blocking=off  timestamp=off  autoconnect=on  errorOnConnection=off
  Inv\* : Product  Inputs=/*  Multiplication=Matrix(*)
  Inv\*1 : Product  Inputs=/*  Multiplication=Matrix(*)
  Inv\*2 : Product  Inputs=/  Multiplication=Matrix(*)
  Product : Product  Multiplication=Matrix(*)
  Selector : Selector  InputPortWidth=12  IndexOptions=Index vector (dialog)  Indices=[4 5 6 ]  OutputSizes=1
  Selector1 : Selector  InputPortWidth=6  IndexOptions=Index vector (dialog)  Indices=[1:3]  OutputSizes=1
  Switch : Switch  Criteria=u2 > Threshold
  Switch6 : Switch  Criteria=u2 > Threshold
  USE_IMU4EST_BASE : Constant  Value=CONFIG.USE_IMU4EST_BASE
  USE_IMU4EST_BASE1 : Constant  Value=CONFIG.CORRECT_NECK_IMU
  fromImuToHomogeousTransformFCN : MATLAB Function  TreatAsAtomicUnit=on
      settings: PermitHierarchicalResolution=ParametersOnly
  holder 1 : WBToolboxLibrary/Utilities/holder 
  holder 2 : WBToolboxLibrary/Utilities/holder 
  imu : WBToolboxLibrary/wholeBodyModel/Kinematics/Forward Kinematics  frameName='imu_frame'  robotName=WBT_robotName  localName=WBT_modelName  wbiFile=WBT_wbiFilename  wbiList=WBT_wbiList
  l_sole_acc : Scope
      settings: TimeRange=60  ShowLegends=on  MaxDataPoints=5000  SaveToWorkspace=off  YMin=-4.47309  YMax=14.2668  SampleTime=-1
  link : WBToolboxLibrary/wholeBodyModel/Kinematics/Forward Kinematics  frameName=link_name  robotName=WBT_robotName  localName=WBT_modelName  wbiFile=WBT_wbiFilename  wbiList=WBT_wbiList
  root_link : WBToolboxLibrary/wholeBodyModel/Kinematics/Forward Kinematics  frameName='root_link'  robotName=WBT_robotName  localName=WBT_modelName  wbiFile=WBT_wbiFilename  wbiList=WBT_wbiList
  w_H_root : Outport
  wires:
  Constant/1 -> Switch/3
  Gain/1 -> Selector1/1
  Switch/1 -> fromImuToHomogeousTransformFCN/6(neck)
  USE_IMU4EST_BASE1/1 -> Switch/2
  Selector1/1 -> Switch/1  "neck"
  Head state/1 -> Gain/1
  Product/1 -> l_sole_acc/1
  Selector/1 -> Product/2  "imu_acce"
  "CoM6D ->  CoMXYZ1"/1 -> Product/1  "l_sole_R_imu"
  Inv\*2/1 -> "CoM6D ->  CoMXYZ1"/1
  holder 2/1 -> fromImuToHomogeousTransformFCN/4(inertial_0)
  holder 1/1 -> fromImuToHomogeousTransformFCN/2(imu_H_link_0)
  root_link/1 -> Inv\*1/2
  qj/1 -> imu/2, link/2, root_link/2
  Constant2/1 -> root_link/1
  fromImuToHomogeousTransformFCN/1(w_H_root) -> Switch6/1
  USE_IMU4EST_BASE/1 -> Switch6/2
  Switch6/1 -> w_H_root/1
  inertial/1 -> fromImuToHomogeousTransformFCN/5(inertial), holder 2/1, Selector/1
  link/1 -> Inv\*1/1, Inv\*/2
  Inv\*1/1 -> fromImuToHomogeousTransformFCN/3(link_H_root), Switch6/3  "link_H_root"
  Constant6/1 -> link/1
  imu/1 -> Inv\*/1
  Inv\*/1 -> fromImuToHomogeousTransformFCN/1(imu_H_link), holder 1/1, Inv\*2/1  "imu_H_link"
  Constant5/1 -> imu/1

== system stepRecovery_compatibility/DesValues/State Machine/visualise inertial/l_sole_H_root_link2/Visualize hom transf4 ==
  H : Inport
  "CoM6D ->  CoMXYZ1" : Selector  NumberOfDimensions=2  InputPortWidth=7  IndexOptions=Index vector (dialog),Index vector (dialog)  Indices=[1 2 3],[1 2 3]  OutputSizes=1,1
  "CoM6D ->  CoMXYZ2" : Selector  NumberOfDimensions=2  InputPortWidth=7  IndexOptions=Index vector (dialog),Index vector (dialog)  Indices=[1 2 3],[4]  OutputSizes=1,1
  Hom : Scope
      settings: TimeRange=auto  ShowLegends=on  MaxDataPoints=5000  SaveToWorkspace=off  SaveName=ScopeData3  YMin=-1.25  YMax=1.25  SampleTime=-1
  R : Scope
      settings: TimeRange=auto  MaxDataPoints=5000  SaveToWorkspace=off  YMin=-0.125  YMax=1.125  SampleTime=-1
  p : Scope
      settings: TimeRange=auto  MaxDataPoints=5000  SaveToWorkspace=off  SaveName=ScopeData2  YMin=-1.00000  YMax=1.00000  SampleTime=-1
  wires:
  "CoM6D ->  CoMXYZ1"/1 -> R/1
  "CoM6D ->  CoMXYZ2"/1 -> p/1
  H/1 -> "CoM6D ->  CoMXYZ2"/1, Hom/1, "CoM6D ->  CoMXYZ1"/1

== system stepRecovery_compatibility/DesValues/State Machine/visualise inertial/l_sole_H_root_link3/Visualize hom transf4 ==
  H : Inport
  "CoM6D ->  CoMXYZ1" : Selector  NumberOfDimensions=2  InputPortWidth=7  IndexOptions=Index vector (dialog),Index vector (dialog)  Indices=[1 2 3],[1 2 3]  OutputSizes=1,1
  "CoM6D ->  CoMXYZ2" : Selector  NumberOfDimensions=2  InputPortWidth=7  IndexOptions=Index vector (dialog),Index vector (dialog)  Indices=[1 2 3],[4]  OutputSizes=1,1
  Hom : Scope
      settings: TimeRange=auto  ShowLegends=on  MaxDataPoints=5000  SaveToWorkspace=off  SaveName=ScopeData3  YMin=-1.25  YMax=1.25  SampleTime=-1
  R : Scope
      settings: TimeRange=auto  MaxDataPoints=5000  SaveToWorkspace=off  YMin=-0.125  YMax=1.125  SampleTime=-1
  p : Scope
      settings: TimeRange=auto  MaxDataPoints=5000  SaveToWorkspace=off  SaveName=ScopeData2  YMin=-1.00000  YMax=1.00000  SampleTime=-1
  wires:
  "CoM6D ->  CoMXYZ1"/1 -> R/1
  "CoM6D ->  CoMXYZ2"/1 -> p/1
  H/1 -> "CoM6D ->  CoMXYZ2"/1, Hom/1, "CoM6D ->  CoMXYZ1"/1

== system stepRecovery_compatibility/DesValues/State Machine Step Recovery/Step Recovery reference generator/Inverse Kinematics/Local inverse kin ==
  Desired Transformation : Inport
  w_H_b : Inport  Port=2
  qj : Inport  Port=3
  Enable : EnablePort
  23-DoFs WBI to YARP : WBToolboxLibrary/Utilities/23-DoFs WBI to YARP
  Inverse Kinematics : WBToolboxLibrary/wholeBodyModel/Kinematics/Inverse Kinematics  baseFrame='l_sole'  endEffFrame='r_sole'  optOption=Full Constraint (Position and Orientation)  robotName=WBT_robotName  localName=WBT_modelName  wbiFile=WBT_wbiFilename  wbiList=WBT_wbiList
  Mux : Mux  Inputs=2
  Terminator{,1..3} (4 alike) : Terminator
  q_legs : Outport
  "q_total " : Outport  Port=2
  wires:
  Desired Transformation/1 -> Inverse Kinematics/1
  23-DoFs WBI to YARP/3 -> Terminator3/1
  Mux/1 -> q_legs/1
  w_H_b/1 -> Inverse Kinematics/2
  23-DoFs WBI to YARP/1 -> Terminator1/1
  23-DoFs WBI to YARP/2 -> Terminator2/1
  qj/1 -> Inverse Kinematics/3
  Inverse Kinematics/1 -> Terminator/1
  Inverse Kinematics/2 -> "q_total "/1, 23-DoFs WBI to YARP/1
  23-DoFs WBI to YARP/4 -> Mux/1
  23-DoFs WBI to YARP/5 -> Mux/2

== system stepRecovery_compatibility/DesValues/State Machine Step Recovery/Step Recovery reference generator/Inverse Kinematics/Pseudo-Inverse kinematics Solver ==
  "lsole_H_rsole " : Inport
  rsole_H_lsole : Inport  Port=2
  q_guess : Inport  Port=3
  NuRef_ikin_ini : Inport  Port=4
  CoMrefsDes : Inport  Port=5
  posturesDes : Inport  Port=6
  constraints : Inport  Port=7
  "w_H_b " : Inport  Port=8
  qj : Inport  Port=9
  Enable : EnablePort
  From guess to q_ikin : Subsystem
  Generate ikin Errors : Subsystem
  constraints1 : InportShadow  Port=7
  ikin visualizer : Subsystem
  ikin_DoubleIntegrator : Subsystem
  ikin_utilities : Subsystem
  q+base : Subsystem
  trajectoryGeneratorCoM : MATLAB Function  TreatAsAtomicUnit=on
      settings: PermitHierarchicalResolution=ParametersOnly
  qjRef_ikin : Outport
  inverseKinRef : Outport  Port=2
  wires:
  Generate ikin Errors/1(iKinFeetCorr) -> trajectoryGeneratorCoM/1(iKinFeetCorr), ikin visualizer/1(Ikin_feetCorr)
  Generate ikin Errors/2(iKinComCorr) -> trajectoryGeneratorCoM/2(iKinComCorr), ikin visualizer/2(Ikin_CoMCorr)
  Generate ikin Errors/4(iKinPostCorr) -> trajectoryGeneratorCoM/4(iKinPostCorr), ikin visualizer/3(Ikin_PostCorr)
  ikin_DoubleIntegrator/2(qRef_ikin) -> ikin_utilities/3(qRef_ikin), Generate ikin Errors/12(qRef_ikin)
  ikin_DoubleIntegrator/1(NuRef_ikin) -> ikin_utilities/4(NuRef_ikin), Generate ikin Errors/11(NuRef_iKin)
  qj/1 -> From guess to q_ikin/3(q0), q+base/1(qj)
  CoMrefsDes/1 -> Generate ikin Errors/1(CoMrefsDes)
  posturesDes/1 -> Generate ikin Errors/2(posturesDes)
  ikin_utilities/1(Jlsole) -> trajectoryGeneratorCoM/5(J_lfoot), Generate ikin Errors/3(Jlfoot)
  ikin_utilities/2(Jrsole) -> trajectoryGeneratorCoM/6(J_rfoot), Generate ikin Errors/4(Jrfoot)
  ikin_utilities/3(JCoM) -> trajectoryGeneratorCoM/7(J_com), Generate ikin Errors/5(JCoM)
  ikin_utilities/4(deltaRFootPos) -> Generate ikin Errors/6(rfootPos)
  ikin_utilities/5(deltaLFootPos) -> Generate ikin Errors/7(lfootPos)
  ikin_utilities/6(CoMPos) -> Generate ikin Errors/8(CoMPos)
  ikin_utilities/7(deltaLFootOri) -> Generate ikin Errors/9(lfootOri)
  ikin_utilities/8(deltaRFootOri) -> Generate ikin Errors/10(rfootOri)
  NuRef_ikin_ini/1 -> ikin_DoubleIntegrator/2(Nu_ikin_init)
  trajectoryGeneratorCoM/1(dNuRef_ikin) -> ikin_DoubleIntegrator/1(dNuRef_ikin)
  constraints/1 -> trajectoryGeneratorCoM/11(constraints)
  ikin_utilities/10(dJlfootNu) -> trajectoryGeneratorCoM/8(dJcNu_lf)
  ikin_utilities/11(dJrfootNu) -> trajectoryGeneratorCoM/9(dJcNu_rf)
  ikin_utilities/12(dJCoMNu) -> trajectoryGeneratorCoM/10(dJ_comNu)
  ikin_DoubleIntegrator/3(inverseKinRef) -> inverseKinRef/1
  ikin_DoubleIntegrator/4(qjRef_ikin) -> qjRef_ikin/1
  q+base/1(qRef_ikin_ini) -> ikin_utilities/5(qRef_ikin_init)
  Generate ikin Errors/3(iKinSoleCorr) -> trajectoryGeneratorCoM/3(iKinSoleCorr), ikin visualizer/4(ikin_sole_Corr)
  "lsole_H_rsole "/1 -> ikin_utilities/1(lsole_H_rsole)
  rsole_H_lsole/1 -> ikin_utilities/2(rsole_H_lsole)
  "w_H_b "/1 -> From guess to q_ikin/2(w_H_b), q+base/2(w_H_b)
  From guess to q_ikin/1(q_ikin_guess) -> ikin_DoubleIntegrator/3(q_guess)
  q_guess/1 -> From guess to q_ikin/4("qGuess ")
  constraints1/1 -> From guess to q_ikin/1(constraints), q+base/3(constraints)
  ikin_utilities/9(cartesian_err) -> Generate ikin Errors/13(cartesian_err)

== system stepRecovery_compatibility/DesValues/State Machine Step Recovery/Step Recovery reference generator/Inverse Kinematics/Remote Inverse Kineamtics ==
  Desired Transformation : Inport
  q(0) : Inport  Port=2
  23-DoFs WBI to YARP1 : WBToolboxLibrary/Utilities/23-DoFs WBI to YARP
  Mux : Mux
  Mux2 : Mux  Inputs=2
  Remote Inverse Kinematics : WBToolboxLibrary/wholeBodyModel/Kinematics/Remote Inverse Kinematics  solverName='/cartesianSolver'  dofs=12  optOption=Full Constraint (Position and Orientation)
  Selector : Selector  InputPortWidth=6  IndexOptions=Index vector (dialog)  Indices=[6 5 4 3 2 1]  OutputSizes=1
  Selector1 : Selector  InputPortWidth=12  IndexOptions=Index vector (dialog)  Indices=[6, 5, 4, 3, 2, 1, 7:12]  OutputSizes=1
  q_legs : Outport
  q_total : Outport  Port=2
  wires:
  Desired Transformation/1 -> Remote Inverse Kinematics/1
  q(0)/1 -> 23-DoFs WBI to YARP1/1
  23-DoFs WBI to YARP1/5 -> Mux2/2
  Mux2/1 -> Remote Inverse Kinematics/2
  23-DoFs WBI to YARP1/4 -> Selector/1
  Selector/1 -> Mux2/1
  Selector1/1 -> Mux/4, q_legs/1
  Remote Inverse Kinematics/1 -> Selector1/1
  23-DoFs WBI to YARP1/1 -> Mux/1
  23-DoFs WBI to YARP1/2 -> Mux/2
  23-DoFs WBI to YARP1/3 -> Mux/3
  Mux/1 -> q_total/1

== system stepRecovery_compatibility/DesValues/State Machine Step Recovery/Step Recovery reference generator/Step Recovery Techniques /Capture Point Computer ==
  r_Cxp : Inport
  COM velocity : Inport  Port=2
  COMx : Inport  Port=3
  w_H_lsole : Inport  Port=4
  w_H_rsole : Inport  Port=5
  "Constraints " : Inport  Port=6
  STATE : Inport  Port=7
  Capture Point : Subsystem
  "Capture Point-Pratt " : Subsystem
  Capture Point-alternative : Subsystem
  Constant : Constant  Value=CONFIG.SR.TECHNIQUE+CONFIG.SR.CP.MODEL+CONFIG.SR.CP.FF
  Constant1 : Constant  Value=zeros(10,1)
  "ICP " : Subsystem
  Out of left foot_CH : Subsystem
  Switch : Switch  Criteria=u2 > Threshold
  w_H_lsole1 : InportShadow  Port=4
  r_CP : Outport
  r_CP1 : Outport  Port=2
  OUT : Outport  Port=3
  Direction : Outport  Port=4
  OUT_REAL : Outport  Port=5
  OUT_CH : Outport  Port=6
  "r_CPratt " : Outport  Port=7
  r_icp : Outport  Port=8
  CoP_ref : Outport  Port=9
  wires:
  r_Cxp/1 -> Capture Point-alternative/2(r_CxP), Capture Point/2(r_CxP)
  COMx/1 -> "ICP "/1(COM position), "Capture Point-Pratt "/3(COMx), Capture Point-alternative/3(COMx), Capture Point/3(COMx)
  COM velocity/1 -> "ICP "/2(COM velocity)
  Capture Point/1("r_CP ") -> r_CP/1
  "ICP "/1(icp) -> r_icp/1, Out of left foot_CH/1(X_global), "Capture Point-Pratt "/4(r_icp), Capture Point-alternative/4(r_icp), Capture Point/4(r_icp)
  Out of left foot_CH/1(OUT_L) -> "Capture Point-Pratt "/5(OUT), Capture Point-alternative/5(OUT), Capture Point/5(OUT)
  Capture Point/2("STEP ") -> OUT/1
  Capture Point-alternative/1("r_CP ") -> r_CP1/1
  Capture Point/3(Direction) -> Direction/1
  Out of left foot_CH/2(OUT_CH) -> Capture Point-alternative/6(OUT_CH), "Capture Point-Pratt "/6(OUT_CH), Capture Point/6(OUT_CH), OUT_CH/1
  "Constraints "/1 -> Out of left foot_CH/2(Constraints)
  Out of left foot_CH/3(OUT_REAL) -> OUT_REAL/1
  w_H_lsole/1 -> Out of left foot_CH/3(w_H_lsole)
  w_H_rsole/1 -> Out of left foot_CH/4(w_H_rsole)
  STATE/1 -> "Capture Point-Pratt "/2(STATE), Capture Point-alternative/1(STATE), Capture Point/1(STATE)
  w_H_lsole1/1 -> "Capture Point-Pratt "/1(w_H_f)
  "Capture Point-Pratt "/1("r_CP ") -> "r_CPratt "/1
  Constant/1 -> Switch/2
  Switch/1 -> CoP_ref/1
  Capture Point/4(CoP_ref) -> Switch/3
  Constant1/1 -> Switch/1

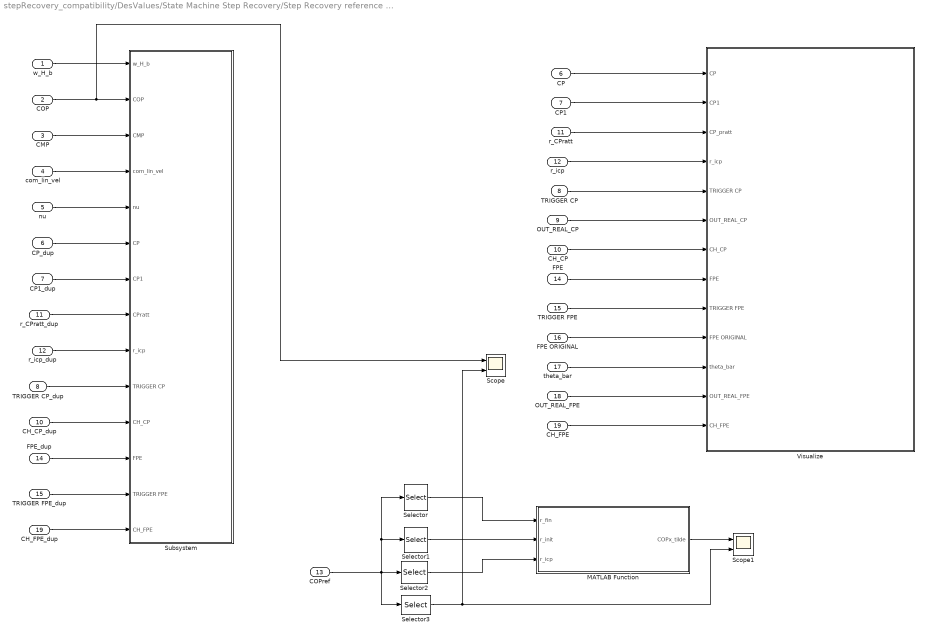
== system stepRecovery_compatibility/DesValues/State Machine Step Recovery/Step Recovery reference generator/Step Recovery Techniques /Dump and Visualize SRT  ==
  w_H_b : Inport
  COP : Inport  Port=2
  CMP : Inport  Port=3
  com_lin_vel : Inport  Port=4
  nu : Inport  Port=5
  CP : Inport  Port=6
  CP1 : Inport  Port=7
  TRIGGER CP : Inport  Port=8
  OUT_REAL_CP : Inport  Port=9
  CH_CP : Inport  Port=10
  "r_CPratt " : Inport  Port=11
  r_icp : Inport  Port=12
  COPref : Inport  Port=13
  FPE : Inport  Port=14
  TRIGGER FPE : Inport  Port=15
  FPE ORIGINAL : Inport  Port=16
  theta_bar : Inport  Port=17
  OUT_REAL_FPE : Inport  Port=18
  CH_FPE : Inport  Port=19
  CH_CP_dup : InportShadow  Port=10
  CH_FPE_dup : InportShadow  Port=19
  CP1_dup : InportShadow  Port=7
  CP_dup : InportShadow  Port=6
  FPE_dup : InportShadow  Port=14
  MATLAB Function : MATLAB Function  TreatAsAtomicUnit=on
      settings: PermitHierarchicalResolution=ParametersOnly
  Scope : Scope  NumInputPorts=2
      settings: TimeRange=auto  MaxDataPoints=5000  SaveToWorkspace=off  SaveName=ScopeData2  YMin=-0.06809~-5  YMax=0.08754~5  SampleTime=-1
  Scope1 : Scope  NumInputPorts=2
      settings: TimeRange=auto  MaxDataPoints=5000  SaveToWorkspace=off  YMin=-0.05032~-5  YMax=0.07122~5  SampleTime=-1
  Selector : Selector  InputPortWidth=10  IndexOptions=Index vector (dialog)  Indices=[1:3]  OutputSizes=1
  Selector1 : Selector  InputPortWidth=10  IndexOptions=Index vector (dialog)  Indices=[4:6]  OutputSizes=1
  Selector2 : Selector  InputPortWidth=10  IndexOptions=Index vector (dialog)  Indices=[7:9]  OutputSizes=1
  Selector3 : Selector  InputPortWidth=10  IndexOptions=Index vector (dialog)  Indices=[10]  OutputSizes=1
  Subsystem : Subsystem
  TRIGGER CP_dup : InportShadow  Port=8
  TRIGGER FPE_dup : InportShadow  Port=15
  "Visualize " : Subsystem
  r_CPratt_dup : InportShadow  Port=11
  r_icp_dup : InportShadow  Port=12
  wires:
  w_H_b/1 -> Subsystem/1(w_H_b)
  COP/1 -> Scope/1, Subsystem/2(COP)
  CMP/1 -> Subsystem/3(CMP)
  com_lin_vel/1 -> Subsystem/4(com_lin_vel)
  nu/1 -> Subsystem/5(nu)
  CP_dup/1 -> Subsystem/6(CP)
  CP1_dup/1 -> Subsystem/7(CP1)
  TRIGGER CP_dup/1 -> Subsystem/10(TRIGGER CP)
  CH_CP_dup/1 -> Subsystem/11(CH_CP)
  FPE_dup/1 -> Subsystem/12(FPE)
  TRIGGER FPE_dup/1 -> Subsystem/13(TRIGGER FPE)
  CH_FPE_dup/1 -> Subsystem/14(CH_FPE)
  CP/1 -> "Visualize "/1(CP)
  CP1/1 -> "Visualize "/2(CP1)
  TRIGGER CP/1 -> "Visualize "/5(TRIGGER CP)
  OUT_REAL_CP/1 -> "Visualize "/6(OUT_REAL_CP)
  CH_CP/1 -> "Visualize "/7(CH_CP)
  FPE/1 -> "Visualize "/8(FPE)
  TRIGGER FPE/1 -> "Visualize "/9(TRIGGER FPE)
  FPE ORIGINAL/1 -> "Visualize "/10(FPE ORIGINAL)
  theta_bar/1 -> "Visualize "/11(theta_bar)
  OUT_REAL_FPE/1 -> "Visualize "/12(OUT_REAL_FPE)
  CH_FPE/1 -> "Visualize "/13(CH_FPE)
  "r_CPratt "/1 -> "Visualize "/3("CP_pratt ")
  r_CPratt_dup/1 -> Subsystem/8("CPratt ")
  r_icp/1 -> "Visualize "/4(r_icp)
  r_icp_dup/1 -> Subsystem/9(r_icp)
  Selector2/1 -> MATLAB Function/3(r_icp)
  Selector1/1 -> MATLAB Function/2(r_init)
  Selector/1 -> MATLAB Function/1(r_fin)
  Selector3/1 -> Scope/2, Scope1/2
  COPref/1 -> Selector3/1, Selector1/1, Selector/1, Selector2/1
  MATLAB Function/1(COPx_tilde) -> Scope1/1
